simulink library "disturbances_lib"  (R2016b)
settings: Solver=VariableStepAuto  StartTime=0.0  StopTime=10.0  RelTol=1e-3
undefined symbols (not defined in the file): fsw_params, sim_params
libraries: aero_drag_lib x1, gravity_lib_2 x1, mag_vec_LS_lib x1, mag_vec_lib x1, solar_pressure_lib x1, sun_vector_lib x1
settings Model: Creator=Taylor  LastModifiedBy=Taylor

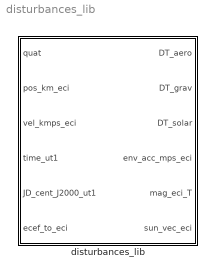
== system disturbances_lib ==
  disturbances_lib : Subsystem

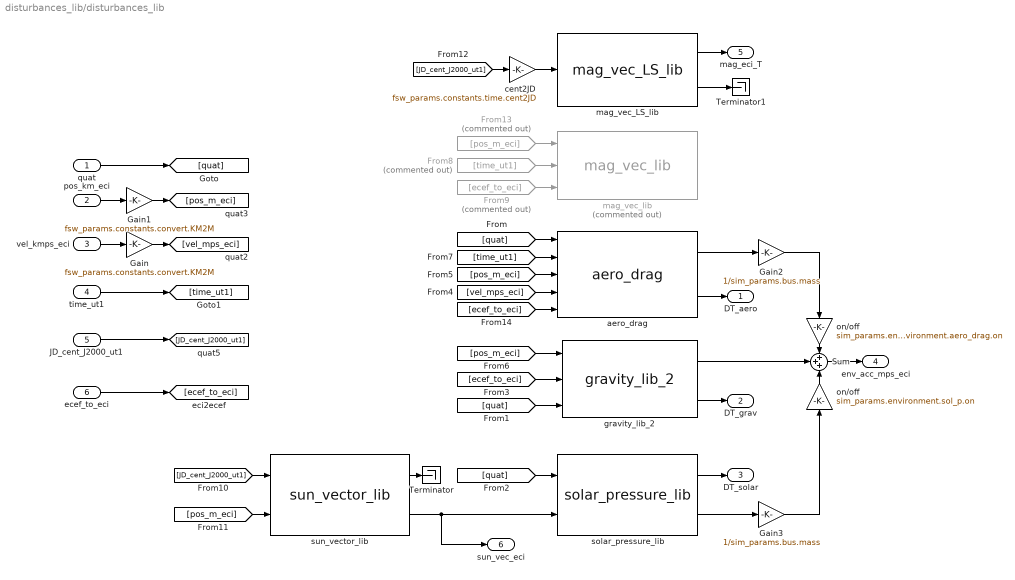
== system disturbances_lib/disturbances_lib ==
  quat : Inport
  pos_km_eci : Inport  Port=2
  vel_kmps_eci : Inport  Port=3
  time_ut1 : Inport  Port=4
  JD_cent_J2000_ut1 : Inport  Port=5
  ecef_to_eci : Inport  Port=6
  From13 : From  Commented=on  GotoTag=pos_m_eci
  From8 : From  Commented=on  GotoTag=time_ut1
  From9 : From  Commented=on  GotoTag=ecef_to_eci
  Gain : Gain  Gain=fsw_params.constants.convert.KM2M
  Gain1 : Gain  Gain=fsw_params.constants.convert.KM2M
  Gain2 : Gain  Gain=1/sim_params.bus.mass
  Gain3 : Gain  Gain=1/sim_params.bus.mass
  Sum : Sum  Inputs=+++
  Terminator : Terminator
  Terminator1 : Terminator
  aero_drag : aero_drag_lib/aero_drag
  cent2JD : Gain  Gain=fsw_params.constants.time.cent2JD
  gravity_lib_2 : gravity_lib_2/gravity_lib_2
  mag_vec_LS_lib : mag_vec_LS_lib/mag_vec_LS_lib
  mag_vec_lib : mag_vec_lib/mag_vec_lib  Commented=on
  on/off : Gain  Gain=sim_params.environment.aero_drag.on
  "on/off " : Gain  Gain=sim_params.environment.sol_p.on
  solar_pressure_lib : solar_pressure_lib/solar_pressure_lib
  sun_vector_lib : sun_vector_lib/sun_vector_lib
  DT_aero : Outport
  DT_grav : Outport  Port=2
  DT_solar : Outport  Port=3
  env_acc_mps_eci : Outport  Port=4
  mag_eci_T : Outport  Port=5
  sun_vec_eci : Outport  Port=6
  wires:
  [quat] -> gravity_lib_2/3
  "on/off "/1 -> Sum/3
  on/off/1 -> Sum/1
  Sum/1 -> env_acc_mps_eci/1
  solar_pressure_lib/1 -> DT_solar/1
  gravity_lib_2/2 -> DT_grav/1
  aero_drag/2 -> DT_aero/1
  From9/1 -> mag_vec_lib/3
  Gain3/1 -> "on/off "/1
  solar_pressure_lib/2 -> Gain3/1
  Gain2/1 -> on/off/1
  aero_drag/1 -> Gain2/1
  gravity_lib_2/1 -> Sum/2
  From13/1 -> mag_vec_lib/1
  sun_vector_lib/2 -> sun_vec_eci/1, solar_pressure_lib/2
  sun_vector_lib/1 -> Terminator/1
  [pos_m_eci] -> sun_vector_lib/2
  [JD_cent_J2000_ut1] -> sun_vector_lib/1
  JD_cent_J2000_ut1/1 -> [JD_cent_J2000_ut1]
  From8/1 -> mag_vec_lib/2
  [time_ut1] -> aero_drag/2
  time_ut1/1 -> [time_ut1]
  [pos_m_eci] -> gravity_lib_2/1
  [pos_m_eci] -> aero_drag/3
  Gain1/1 -> [pos_m_eci]
  pos_km_eci/1 -> Gain1/1
  [vel_mps_eci] -> aero_drag/4
  Gain/1 -> [vel_mps_eci]
  vel_kmps_eci/1 -> Gain/1
  [ecef_to_eci] -> gravity_lib_2/2
  [quat] -> solar_pressure_lib/1
  [quat] -> aero_drag/1
  ecef_to_eci/1 -> [ecef_to_eci]
  quat/1 -> [quat]
  [ecef_to_eci] -> aero_drag/5
  mag_vec_LS_lib/1 -> mag_eci_T/1
  mag_vec_LS_lib/2 -> Terminator1/1
  [JD_cent_J2000_ut1] -> cent2JD/1
  cent2JD/1 -> mag_vec_LS_lib/1
